simulink model "untitled"  (R2015a)
settings: Solver=FixedStepDiscrete  SolverMode=SingleTasking  StartTime=0.0  StopTime=10.0  FixedStep=1e-3  RelTol=1e-3
libraries: mbed_spi_several x1
settings Model: Creator=oh  LastModifiedBy=oh
settings OptimizationCC: OptimizeModelRefInitCode=on  LifeSpan=1
settings HardwareCC: ProdLargestAtomicInteger=Long  ProdLargestAtomicFloat=Double  ProdEndianess=LittleEndian  ProdHWDeviceType=ARM Compatible->ARM Cortex
settings RTWCC: SystemTargetFile=mbed.tlc  TemplateMakefile=mbed.tmf  Description=Mbed Target (Embedded Target)  TargetLang=C++
settings CodeAppCC: IgnoreCustomStorageClasses=off
settings STFCustomTargetCC: CombineOutputUpdateFcns=on  SupportContinuousTime=off  SupportVariableSizeSignals=off  SystemTargetFile=mbed.tlc
settings ERTTargetCC: SupportContinuousTime=off  SupportVariableSizeSignals=off  ERTCustomFileTemplate=mbed_file_process.tlc

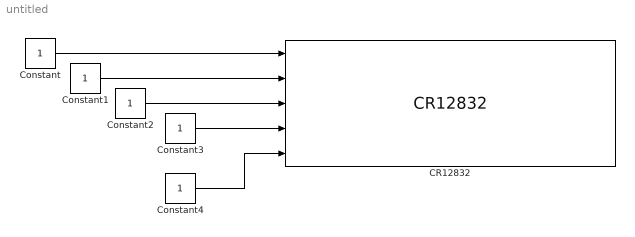
== system untitled ==
  CR12832 : mbed_spi_several/CR12832  TypeOfInputs1={'uint8' 'int8' 'int8'}  NumberOfInputs1=3  Row1='ABC %d %d %d'  TypeOfInputs2={'single'}  NumberOfInputs2=1  Row2='test2 %f'  TypeOfInputs3={'single'}  NumberOfInputs3=1  Row3='test3 %f'  BufferSize=100  SpiPort=1  CsPort=A  CsPin=0  SampleTime=-1
  Constant{,1..4} (5 alike) : Constant  OutDataTypeStr=Inherit: Inherit via back propagation
  wires:
  Constant3/1 -> CR12832/4
  Constant2/1 -> CR12832/3
  Constant1/1 -> CR12832/2
  Constant/1 -> CR12832/1
  Constant4/1 -> CR12832/5
